simulink library "to_DCM"  (R2020b)
settings: Solver=VariableStepAuto  StartTime=0.0  StopTime=10.0  RelTol=1e-3
libraries: mat_3x3 x1
settings Model: Creator=whitehole  LastModifiedBy=whitehole

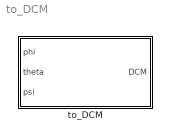
== system to_DCM ==
  to_DCM : Subsystem

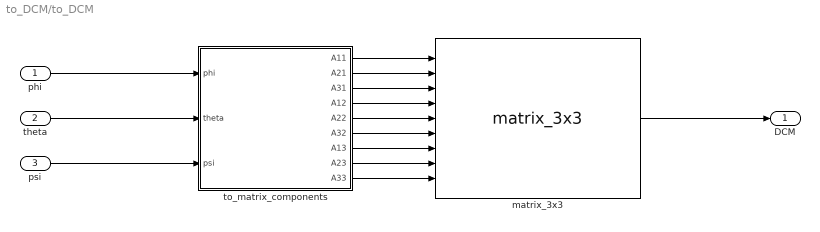
== system to_DCM/to_DCM ==
  phi : Inport
  theta : Inport  Port=2
  psi : Inport  Port=3
  matrix_3x3 : mat_3x3/matrix_3x3  SystemSampleTime=-1  VariantActivationTime=update diagram  Latency=0  AutoFrameSizeCalculation=off
  to_matrix_components : Subsystem
  DCM : Outport
  wires:
  theta/1 -> to_matrix_components/2(theta)
  to_matrix_components/4(A12) -> matrix_3x3/4
  to_matrix_components/9(A33) -> matrix_3x3/9
  to_matrix_components/2(A21) -> matrix_3x3/2
  to_matrix_components/5(A22) -> matrix_3x3/5
  to_matrix_components/7(A13) -> matrix_3x3/7
  psi/1 -> to_matrix_components/3(psi)
  to_matrix_components/3(A31) -> matrix_3x3/3
  matrix_3x3/1 -> DCM/1
  phi/1 -> to_matrix_components/1(phi)
  to_matrix_components/1(A11) -> matrix_3x3/1
  to_matrix_components/6(A32) -> matrix_3x3/6
  to_matrix_components/8(A23) -> matrix_3x3/8

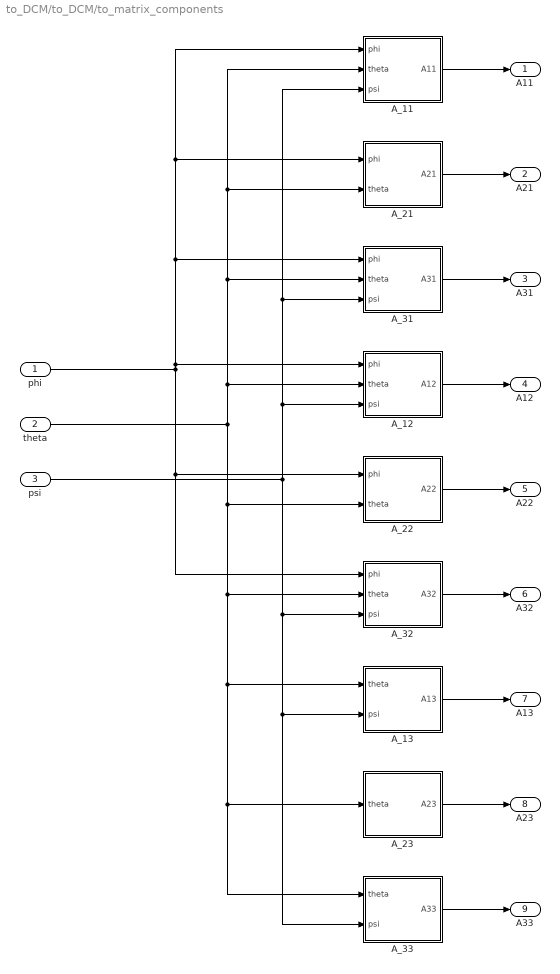
== system to_DCM/to_DCM/to_matrix_components ==
  phi : Inport
  theta : Inport  Port=2
  psi : Inport  Port=3
  A_11 : Subsystem
  A_12 : Subsystem
  A_13 : Subsystem
  A_21 : Subsystem
  A_22 : Subsystem
  A_23 : Subsystem
  A_31 : Subsystem
  A_32 : Subsystem
  A_33 : Subsystem
  A11 : Outport
  A21 : Outport  Port=2
  A31 : Outport  Port=3
  A12 : Outport  Port=4
  A22 : Outport  Port=5
  A32 : Outport  Port=6
  A13 : Outport  Port=7
  A23 : Outport  Port=8
  A33 : Outport  Port=9
  wires:
  A_11/1(A11) -> A11/1
  A_21/1(A21) -> A21/1
  A_31/1(A31) -> A31/1
  A_12/1(A12) -> A12/1
  A_22/1(A22) -> A22/1
  A_13/1(A13) -> A13/1
  A_23/1(A23) -> A23/1
  A_33/1(A33) -> A33/1
  A_32/1(A32) -> A32/1
  phi/1 -> A_32/1(phi), A_22/1(phi), A_11/1(phi), A_21/1(phi), A_31/1(phi), A_12/1(phi)
  theta/1 -> A_12/2(theta), A_31/2(theta), A_11/2(theta), A_21/2(theta), A_33/1(theta), A_23/1(theta), A_13/1(theta), A_32/2(theta), A_22/2(theta)
  psi/1 -> A_12/3(psi), A_31/3(psi), A_11/3(psi), A_33/2(psi), A_13/2(psi), A_32/3(psi)

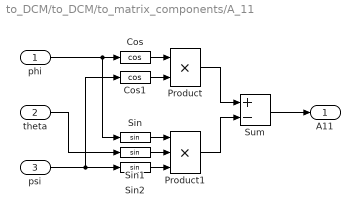
== system to_DCM/to_DCM/to_matrix_components/A_11 ==
  phi : Inport
  theta : Inport  Port=2
  psi : Inport  Port=3
  Cos : Trigonometry  Operator=cos
  Cos1 : Trigonometry  Operator=cos
  Product : Product
  Product1 : Product  Inputs=3
  Sin : Trigonometry
  Sin1 : Trigonometry
  Sin2 : Trigonometry
  Sum : Sum  Inputs=+-
  A11 : Outport
  wires:
  Sum/1 -> A11/1
  Cos/1 -> Product/1
  Cos1/1 -> Product/2
  Sin1/1 -> Product1/2
  Sin2/1 -> Product1/3
  Sin/1 -> Product1/1
  Product/1 -> Sum/1
  Product1/1 -> Sum/2
  psi/1 -> Cos1/1, Sin2/1
  phi/1 -> Cos/1, Sin/1
  theta/1 -> Sin1/1

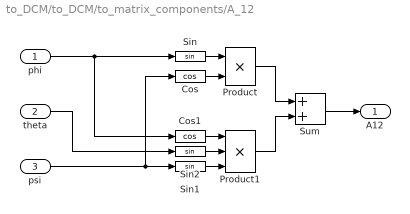
== system to_DCM/to_DCM/to_matrix_components/A_12 ==
  phi : Inport
  theta : Inport  Port=2
  psi : Inport  Port=3
  Cos : Trigonometry  Operator=cos
  Cos1 : Trigonometry  Operator=cos
  Product : Product
  Product1 : Product  Inputs=3
  Sin : Trigonometry
  Sin1 : Trigonometry
  Sin2 : Trigonometry
  Sum : Sum
  A12 : Outport
  wires:
  Product1/1 -> Sum/2
  Sum/1 -> A12/1
  Product/1 -> Sum/1
  psi/1 -> Cos/1, Sin1/1
  phi/1 -> Sin/1, Cos1/1
  Cos/1 -> Product/2
  Sin/1 -> Product/1
  theta/1 -> Sin2/1
  Cos1/1 -> Product1/1
  Sin2/1 -> Product1/2
  Sin1/1 -> Product1/3

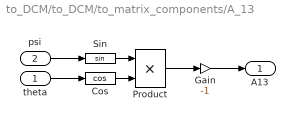
== system to_DCM/to_DCM/to_matrix_components/A_13 ==
  theta : Inport
  psi : Inport  Port=2
  Cos : Trigonometry  Operator=cos
  Gain : Gain  Gain=-1
  Product : Product
  Sin : Trigonometry
  A13 : Outport
  wires:
  Sin/1 -> Product/1
  Cos/1 -> Product/2
  Product/1 -> Gain/1
  Gain/1 -> A13/1
  psi/1 -> Sin/1
  theta/1 -> Cos/1

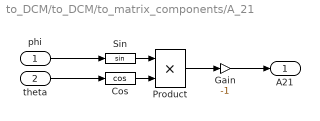
== system to_DCM/to_DCM/to_matrix_components/A_21 ==
  phi : Inport
  theta : Inport  Port=2
  Cos : Trigonometry  Operator=cos
  Gain : Gain  Gain=-1
  Product : Product
  Sin : Trigonometry
  A21 : Outport
  wires:
  Product/1 -> Gain/1
  Gain/1 -> A21/1
  Cos/1 -> Product/2
  Sin/1 -> Product/1
  phi/1 -> Sin/1
  theta/1 -> Cos/1

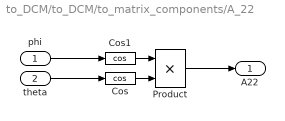
== system to_DCM/to_DCM/to_matrix_components/A_22 ==
  phi : Inport
  theta : Inport  Port=2
  Cos : Trigonometry  Operator=cos
  Cos1 : Trigonometry  Operator=cos
  Product : Product
  A22 : Outport
  wires:
  Cos1/1 -> Product/1
  theta/1 -> Cos/1
  Cos/1 -> Product/2
  phi/1 -> Cos1/1
  Product/1 -> A22/1

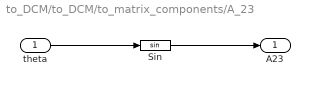
== system to_DCM/to_DCM/to_matrix_components/A_23 ==
  theta : Inport
  Sin : Trigonometry
  A23 : Outport
  wires:
  theta/1 -> Sin/1
  Sin/1 -> A23/1

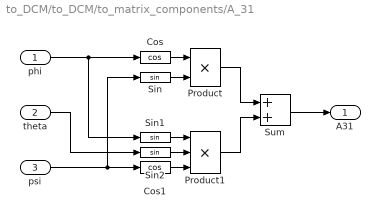
== system to_DCM/to_DCM/to_matrix_components/A_31 ==
  phi : Inport
  theta : Inport  Port=2
  psi : Inport  Port=3
  Cos : Trigonometry  Operator=cos
  Cos1 : Trigonometry  Operator=cos
  Product : Product
  Product1 : Product  Inputs=3
  Sin : Trigonometry
  Sin1 : Trigonometry
  Sin2 : Trigonometry
  Sum : Sum
  A31 : Outport
  wires:
  Sum/1 -> A31/1
  Product1/1 -> Sum/2
  Product/1 -> Sum/1
  psi/1 -> Sin/1, Cos1/1
  phi/1 -> Sin1/1, Cos/1
  Sin/1 -> Product/2
  Cos/1 -> Product/1
  theta/1 -> Sin2/1
  Cos1/1 -> Product1/3
  Sin2/1 -> Product1/2
  Sin1/1 -> Product1/1

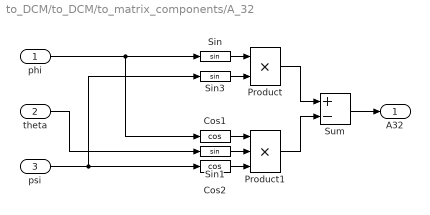
== system to_DCM/to_DCM/to_matrix_components/A_32 ==
  phi : Inport
  theta : Inport  Port=2
  psi : Inport  Port=3
  Cos1 : Trigonometry  Operator=cos
  Cos2 : Trigonometry  Operator=cos
  Product : Product
  Product1 : Product  Inputs=3
  Sin : Trigonometry
  Sin1 : Trigonometry
  Sin3 : Trigonometry
  Sum : Sum  Inputs=+-
  A32 : Outport
  wires:
  Cos1/1 -> Product1/1
  Sin3/1 -> Product/2
  Sum/1 -> A32/1
  Product1/1 -> Sum/2
  Product/1 -> Sum/1
  Sin/1 -> Product/1
  phi/1 -> Cos1/1, Sin/1
  psi/1 -> Sin3/1, Cos2/1
  theta/1 -> Sin1/1
  Cos2/1 -> Product1/3
  Sin1/1 -> Product1/2

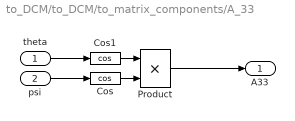
== system to_DCM/to_DCM/to_matrix_components/A_33 ==
  theta : Inport
  psi : Inport  Port=2
  Cos : Trigonometry  Operator=cos
  Cos1 : Trigonometry  Operator=cos
  Product : Product
  A33 : Outport
  wires:
  Cos1/1 -> Product/1
  psi/1 -> Cos/1
  Cos/1 -> Product/2
  theta/1 -> Cos1/1
  Product/1 -> A33/1
